simulink library "calc_G_Fgrav"  (R2020a)
settings: Solver=VariableStepAuto  StartTime=0.0  StopTime=10.0  RelTol=1e-3
settings Model: Creator=Ayaz  LastModifiedBy=Ayaz

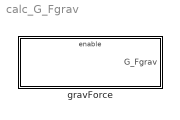
== system calc_G_Fgrav ==
  gravForce : Subsystem  TreatAsAtomicUnit=on  mask{mass=0, gravAccel=9.81}
      mask prompts: mass "Kite mass [kg]"; gravAccel "Gravitational acceleration [m/s^2]"

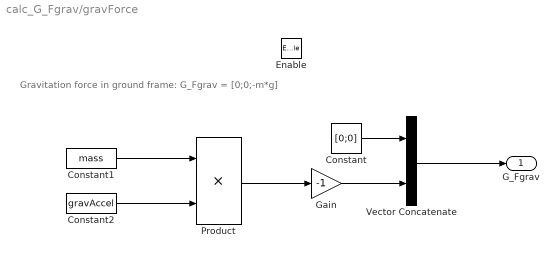
== system calc_G_Fgrav/gravForce ==
  note: Gravitation force in ground frame: G_Fgrav = [0;0;-m*g]
  Enable : EnablePort
  Constant : Constant  Value=[0;0]  VectorParams1D=off
  Constant1 : Constant  Value=mass
  Constant2 : Constant  Value=gravAccel  VectorParams1D=off
  Gain : Gain  Gain=-1
  Product : Product
  Vector Concatenate : Concatenate
  G_Fgrav : Outport
  wires:
  Constant1/1 -> Product/1
  Constant2/1 -> Product/2
  Product/1 -> Gain/1
  Gain/1 -> Vector Concatenate/2
  Constant/1 -> Vector Concatenate/1
  Vector Concatenate/1 -> G_Fgrav/1
